simulink model "CruiseControl_PI_Controller"  (R2026a)
settings: Solver=ode45  StopTime=120  MaxStep=0.01
settings Model: Creator=YASHRK  LastModifiedBy=YASHRK

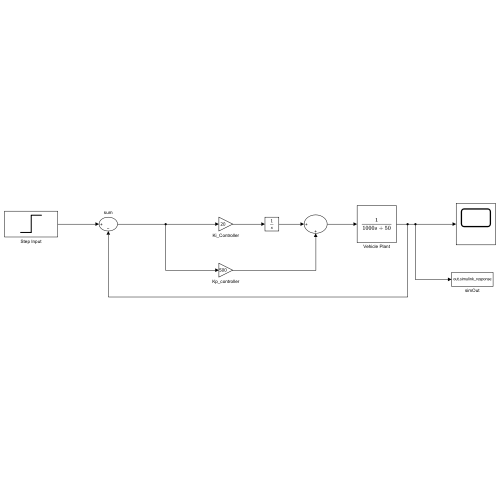
[thumbnail: Simulink's stored preview of the top-level diagram]
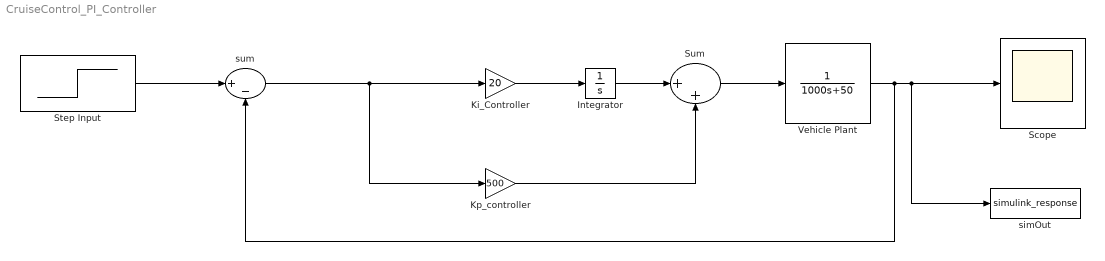
== system CruiseControl_PI_Controller ==
  Integrator : Integrator
  Ki_Controller : Gain  Gain=20
  Kp_controller : Gain  Gain=500
  Scope : Scope
      settings: ActiveDisplayYMinimum=0.22341124678240531  ActiveDisplayYMaximum=1.0713832884149355
  Step Input : Step  Time=0  SampleTime=0
  Sum : Sum  Inputs=|++
  Vehicle Plant : TransferFcn  Denominator=[1000 50]
  simOut : ToWorkspace  VariableName=simulink_response  SaveFormat=Structure With Time  SampleTime=-1
  sum : Sum  Inputs=|+-
  wires:
  Step Input/1 -> sum/1
  Vehicle Plant/1 -> simOut/1, Scope/1, sum/2
  Sum/1 -> Vehicle Plant/1
  Ki_Controller/1 -> Integrator/1
  sum/1 -> Ki_Controller/1, Kp_controller/1
  Kp_controller/1 -> Sum/2
  Integrator/1 -> Sum/1
